simulink model "vrtut2"  (Simulink 6.0)
settings: Solver=ode45  StartTime=0.0  StopTime=15  RelTol=1e-3
libraries: aerospace x1, vrlib x1
settings Model: CovMetricSettings=d  Creator=Straka  LastModifiedBy=Houska  ExtModeTrigMode=oneshot  ExtModeArmWhenConnect=off
settings DataIOCC: SaveOutput=off  SaveTime=off  SignalLoggingName=logsOut
settings OptimizationCC: BlockReduction=off  BooleanDataType=off
settings DebuggingCC: CheckExecutionContextPreStartOutputMsg=on  CheckExecutionContextRuntimeOutputMsg=on  SolverPrmCheckMsg=none
settings HardwareCC: TargetUnknown=on
settings ModelReferenceCC: UpdateModelReferenceTargets=IfOutOfDate
settings GRTTargetCC: LifeSpan=inf
settings SFSimCC: SFSimApplyToAllLibs=on  SFSimBuildMode=Incremental

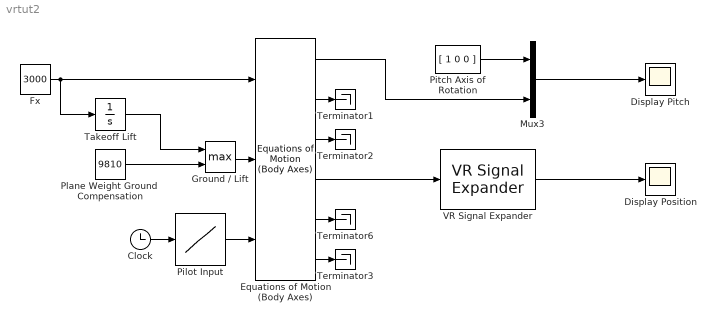
== system vrtut2 ==
  " Equations of Motion (Body Axes)" : aerospace/3DoF Equations of Motion / Equations of Motion (Body Axes)  v_ini=0  theta_ini=0  alpha_ini=0  q_ini=0  pos_ini=[0 0]  mass=1000  Iyy=1000  g=-9.81
  Clock : Clock
      settings: Decimation=10
  Display Pitch : Scope
      settings: YMin=-2  YMax=2
  Display Position : Scope
      settings: YMax=120
  Fx : Constant  Value=3000
  Ground / Lift : MinMax  Function=max  Inputs=2  SaturateOnIntegerOverflow=on  InputSameDT=on
  Mux3 : Mux  Inputs=2
  Pilot Input : Lookup  DialogController=Simulink.DDGSource  InputValues=[0 1 2 8 9 15]  OutputValues=[0 0 -20 20 0 0]  SaturateOnIntegerOverflow=on
  Pitch Axis of Rotation : Constant  Value=[ 1 0 0 ]
  Plane Weight Ground  Compensation : Constant  Value=9810
  Takeoff Lift : Integrator  LimitOutput=on  UpperSaturationLimit=11000  LowerSaturationLimit=-Inf
  Terminator{1..3,6} (4 alike) : Terminator
  VR Signal Expander : vrlib/VR Signal Expander  outwidth=3  outidx=[3 2]
  wires:
  Pitch Axis of Rotation/1 -> Mux3/1
  " Equations of Motion (Body Axes)"/1 -> Mux3/2
  " Equations of Motion (Body Axes)"/2 -> Terminator1/1
  " Equations of Motion (Body Axes)"/3 -> Terminator2/1
  Ground / Lift/1 -> " Equations of Motion (Body Axes)"/2
  Takeoff Lift/1 -> Ground / Lift/1
  Plane Weight Ground  Compensation/1 -> Ground / Lift/2
  Clock/1 -> Pilot Input/1
  Pilot Input/1 -> " Equations of Motion (Body Axes)"/3
  Fx/1 -> " Equations of Motion (Body Axes)"/1, Takeoff Lift/1
  VR Signal Expander/1 -> Display Position/1
  Mux3/1 -> Display Pitch/1
  " Equations of Motion (Body Axes)"/6 -> Terminator3/1
  " Equations of Motion (Body Axes)"/5 -> Terminator6/1
  " Equations of Motion (Body Axes)"/4 -> VR Signal Expander/1
